simulink model "ex3_3"  (R2021a)
settings: Solver=VariableStepAuto  StartTime=0.0  StopTime=100  RelTol=1e-3
values from neighbouring files (symbols this model uses):
  b = 0.001    [parameters.m]
  D = diag([d,d,d].')    [uas_parameters_mod.m]
  g_acc = 9.81    [parameters.m]    (also in uas_parameters_mod.m)
  I = [Ix 0 0; 0 Iy 0; 0 0 Iz]    [parameters.m]    (also in uas_parameters_mod.m)
  invI = inv(I)    [uas_parameters_mod.m]
  Ix = 3*exp(-3)    [parameters.m]    (also in uas_parameters_mod.m = 3*exp(-6))
  Iy = 3*exp(-3)    [parameters.m]    (also in uas_parameters_mod.m = 3*exp(-6))
  Iz = 5*exp(-6)    [parameters.m]    (also in uas_parameters_mod.m = 1*exp(-5))
  k = 0.01    [parameters.m]
  Kd__y = -0.075*K__y*T__y*45    [uas_parameters_mod.m]
  Kd_p = -0.075*K_p*T_p*17    (= 0.7919025)    [uas_parameters_mod.m]
  Kd_r = -0.075*K_r*T_r*6.2    (= 0.79515)    [uas_parameters_mod.m]
  Kd_x = -0.075*K_x*T_x*45    (= 0.022325972625)    [uas_parameters_mod.m]
  Kd_y = -0.075*K_y*T_y*7    (= 0.937125)    [uas_parameters_mod.m]
  Kd_z = -65    [uas_parameters_mod.m]
  Ki__y = 0    [uas_parameters_mod.m]
  Ki_p = 1.2*K_p/T_p*1.2    (= -0.000231846723555)    [uas_parameters_mod.m]
  Ki_r = 1.2*K_r/T_r*0.3    (= -0.00118421052632)    [uas_parameters_mod.m]
  Ki_y = 1.2*K_y/T_y*0.1    (= -0.000378151260504)    [uas_parameters_mod.m]
  Ki_z = 0.01    [uas_parameters_mod.m]
  Kp__y = 0.6*K__y*15    [uas_parameters_mod.m]
  Kp_p = 0.6*K_p*40    (= -0.24)    [uas_parameters_mod.m]
  Kp_r = 0.6*K_r*6    (= -0.27)    [uas_parameters_mod.m]
  Kp_x = 0.6*K_x*15    (= -0.002097)    [uas_parameters_mod.m]
  Kp_y = 0.6*K_y*10    (= -0.45)    [uas_parameters_mod.m]
  Kp_z = 20    [uas_parameters_mod.m]
  L = 0.225    [parameters.m]    (also in uas_parameters_mod.m)
  m = 0.5    [parameters.m]    (also in uas_parameters_mod.m)
  mg = [0; 0; -m*9.81]    [uas_parameters_mod.m]
libraries: slctrlblks x1, vrlib x1
settings Model: Creator=filippo  LastModifiedBy=filippo

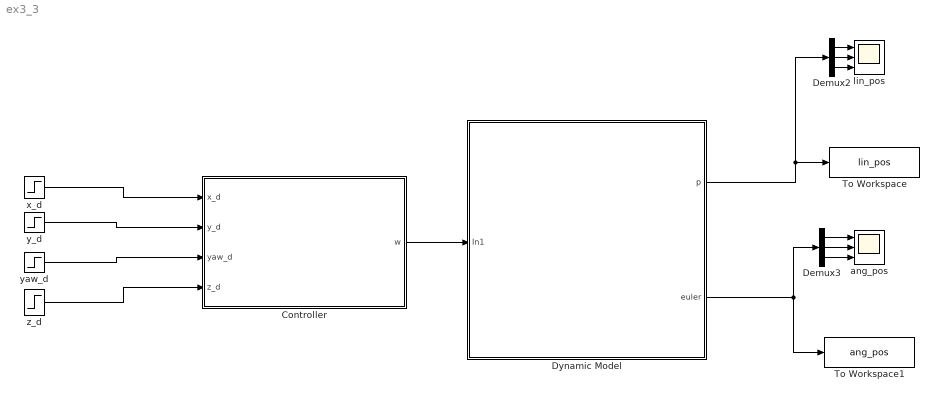
== system ex3_3 ==
  Controller : Subsystem
  Demux2 : Demux  Outputs=3
  Demux3 : Demux  Outputs=3
  Dynamic Model : Subsystem
  To Workspace : ToWorkspace  VariableName=lin_pos  SaveFormat=Timeseries  SampleTime=-1
  To Workspace1 : ToWorkspace  VariableName=ang_pos  SaveFormat=Timeseries  SampleTime=-1
  ang_pos : Scope  NumInputPorts=3
  lin_pos : Scope  NumInputPorts=3
  x_d : Step  SampleTime=0
  y_d : Step  After=0  SampleTime=0
  yaw_d : Step  After=0  SampleTime=0
  z_d : Step  After=0  SampleTime=0
  wires:
  Dynamic Model/2(euler) -> Demux3/1, To Workspace1/1
  Dynamic Model/1(p) -> Demux2/1, To Workspace/1
  Demux2/1 -> lin_pos/1
  Demux3/2 -> ang_pos/2
  Demux2/3 -> lin_pos/3
  Demux2/2 -> lin_pos/2
  Demux3/3 -> ang_pos/3
  Demux3/1 -> ang_pos/1
  Controller/1(w) -> Dynamic Model/1(In1)
  z_d/1 -> Controller/4(z_d)
  x_d/1 -> Controller/1(x_d)
  yaw_d/1 -> Controller/3(yaw_d)
  y_d/1 -> Controller/2(y_d)

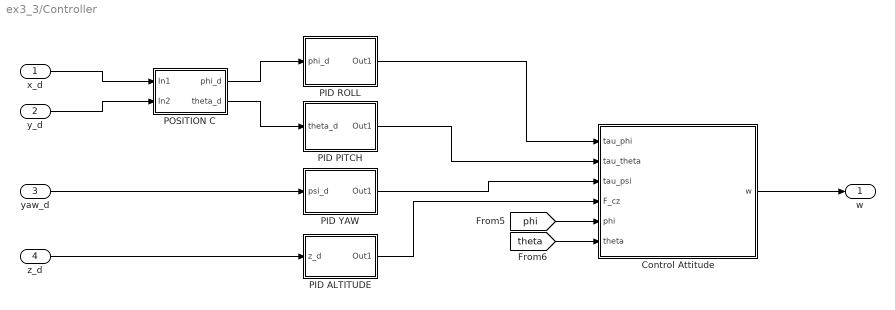
== system ex3_3/Controller ==
  x_d : Inport
  y_d : Inport  Port=2
  yaw_d : Inport  Port=3
  z_d : Inport  Port=4
  Control Attitude : MATLAB Function  TreatAsAtomicUnit=on
  PID ALTITUDE : Subsystem
  PID PITCH : Subsystem
  PID ROLL : Subsystem
  PID YAW : Subsystem
  POSITION C : Subsystem
  w : Outport
  wires:
  PID YAW/1(Out1) -> Control Attitude/3(tau_psi)
  [theta] -> Control Attitude/6(theta)
  PID ROLL/1(Out1) -> Control Attitude/1(tau_phi)
  [phi] -> Control Attitude/5(phi)
  PID ALTITUDE/1(Out1) -> Control Attitude/4(F_cz)
  PID PITCH/1(Out1) -> Control Attitude/2(tau_theta)
  Control Attitude/1(w) -> w/1
  POSITION C/1(phi_d) -> PID ROLL/1(phi_d)
  POSITION C/2(theta_d) -> PID PITCH/1(theta_d)
  x_d/1 -> POSITION C/1(In1)
  y_d/1 -> POSITION C/2(In2)
  z_d/1 -> PID ALTITUDE/1(z_d)
  yaw_d/1 -> PID YAW/1(psi_d)

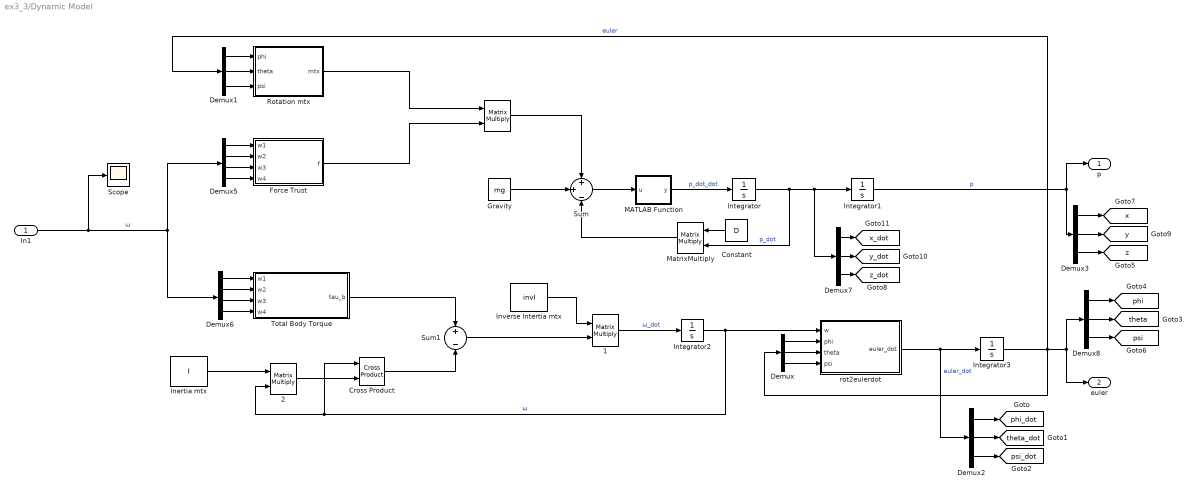
== system ex3_3/Dynamic Model ==
  In1 : Inport
  " " : Product  Multiplication=Matrix(*)
  " 1" : Product  Multiplication=Matrix(*)
  " 2" : Product  Multiplication=Matrix(*)
  Constant : Constant  Value=D
  Cross Product : vrlib/Utilities/Cross Product
  Demux{,1..3,7..8} (6 alike) : Demux  Outputs=3
  Demux5 : Demux
  Demux6 : Demux
  Force Trust : MATLAB Function  TreatAsAtomicUnit=on
  Gravity : Constant  Value=mg  VectorParams1D=off
  Inertia mtx : Constant  Value=I  VectorParams1D=off
  Integrator{,1..3} (4 alike) : Integrator
  Inverse Intertia mtx : Constant  Value=invI
  MATLAB Function : MATLAB Function  TreatAsAtomicUnit=on
  MatrixMultiply : Product  Multiplication=Matrix(*)
  Rotation mtx : MATLAB Function  TreatAsAtomicUnit=on
  Scope : Scope
  Sum : Sum  Inputs=+|+|-
  Sum1 : Sum  Inputs=+|-
  Total Body Torque : MATLAB Function  TreatAsAtomicUnit=on
  rot2eulerdot : MATLAB Function  TreatAsAtomicUnit=on
  p : Outport
  euler : Outport  Port=2
  tag scope: phi=global, phi_dot=global, psi=global, psi_dot=global, theta=global, theta_dot=global, x=global, x_dot=global, y=global, y_dot=global, z=global, z_dot=global
  wires:
  " "/1 -> Sum/1
  Sum/1 -> MATLAB Function/1(u)
  " 2"/1 -> Cross Product/2
  Rotation mtx/1(mtx) -> " "/1
  Demux5/4 -> Force Trust/4(w4)
  Demux1/3 -> Rotation mtx/3(psi)
  Demux5/2 -> Force Trust/2(w2)
  Gravity/1 -> Sum/2
  Demux1/1 -> Rotation mtx/1(phi)
  Demux1/2 -> Rotation mtx/2(theta)
  Demux6/4 -> Total Body Torque/4(w4)
  Demux/2 -> rot2eulerdot/3(theta)
  rot2eulerdot/1(euler_dot) -> Demux2/1, Integrator3/1  "euler_dot"
  Force Trust/1(f) -> " "/2
  Integrator3/1 -> Demux1/1, Demux/1, euler/1, Demux8/1  "euler"
  Demux/1 -> rot2eulerdot/2(phi)
  Demux5/3 -> Force Trust/3(w3)
  Demux6/1 -> Total Body Torque/1(w1)
  In1/1 -> Scope/1, Demux6/1, Demux5/1  "ω"
  Integrator2/1 -> Cross Product/1, " 2"/2, rot2eulerdot/1(w)  "ω"
  Demux6/3 -> Total Body Torque/3(w3)
  Demux/3 -> rot2eulerdot/4(psi)
  Demux5/1 -> Force Trust/1(w1)
  Demux6/2 -> Total Body Torque/2(w2)
  Demux2/1 -> [phi_dot]
  Demux2/3 -> [psi_dot]
  Demux2/2 -> [theta_dot]
  Demux3/3 -> [z]
  Integrator1/1 -> Demux3/1, p/1  "p"
  Integrator/1 -> MatrixMultiply/2, Demux7/1, Integrator1/1  "p_dot"
  Demux7/3 -> [z_dot]
  Demux3/1 -> [x]
  Demux3/2 -> [y]
  Demux7/1 -> [x_dot]
  Demux7/2 -> [y_dot]
  Demux8/1 -> [phi]
  Demux8/2 -> [theta]
  Demux8/3 -> [psi]
  Total Body Torque/1(tau_b) -> Sum1/1
  Cross Product/1 -> Sum1/2
  " 1"/1 -> Integrator2/1  "ω_dot"
  Sum1/1 -> " 1"/2
  Inertia mtx/1 -> " 2"/1
  Inverse Intertia mtx/1 -> " 1"/1
  MATLAB Function/1(y) -> Integrator/1  "p_dot_dot"
  Constant/1 -> MatrixMultiply/1
  MatrixMultiply/1 -> Sum/3

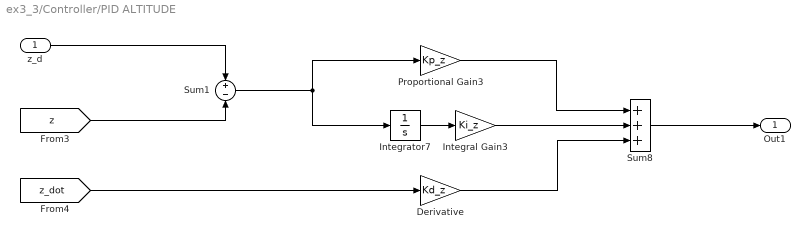
== system ex3_3/Controller/PID ALTITUDE ==
  z_d : Inport
  "Derivative " : Gain  Gain=Kd_z
  Integral Gain3 : Gain  Gain=Ki_z
  Integrator7 : Integrator
  Proportional Gain3 : Gain  Gain=Kp_z
  Sum1 : Sum  Inputs=+|-
  Sum8 : Sum  Inputs=+++
  Out1 : Outport
  wires:
  [z] -> Sum1/2
  "Derivative "/1 -> Sum8/3
  [z_dot] -> "Derivative "/1
  Sum1/1 -> Integrator7/1, Proportional Gain3/1
  Integral Gain3/1 -> Sum8/2
  Integrator7/1 -> Integral Gain3/1
  z_d/1 -> Sum1/1
  Proportional Gain3/1 -> Sum8/1
  Sum8/1 -> Out1/1

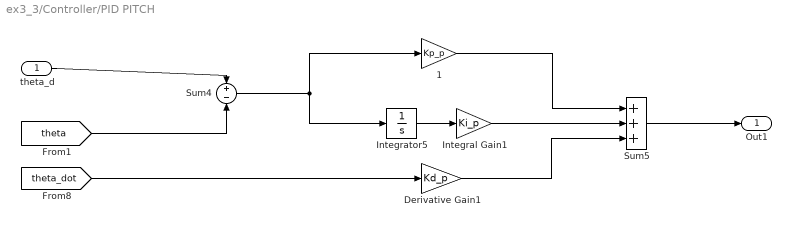
== system ex3_3/Controller/PID PITCH ==
  theta_d : Inport
  " 1" : Gain  Gain=Kp_p
  Derivative Gain1 : Gain  Gain=Kd_p
  Integral Gain1 : Gain  Gain=Ki_p
  Integrator5 : Integrator
  Sum4 : Sum  Inputs=+|-
  Sum5 : Sum  Inputs=+++
  Out1 : Outport
  wires:
  [theta_dot] -> Derivative Gain1/1
  theta_d/1 -> Sum4/1
  Integral Gain1/1 -> Sum5/2
  [theta] -> Sum4/2
  " 1"/1 -> Sum5/1
  Sum4/1 -> " 1"/1, Integrator5/1
  Integrator5/1 -> Integral Gain1/1
  Derivative Gain1/1 -> Sum5/3
  Sum5/1 -> Out1/1

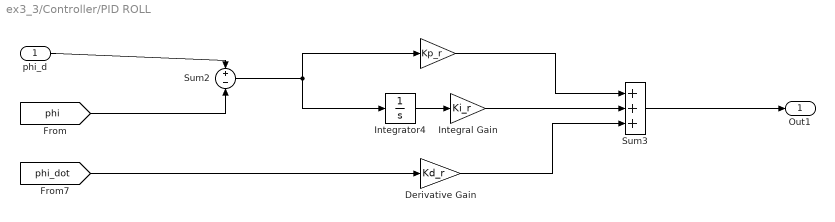
== system ex3_3/Controller/PID ROLL ==
  phi_d : Inport
  " " : Gain  Gain=Kp_r
  Derivative Gain : Gain  Gain=Kd_r
  Integral Gain : Gain  Gain=Ki_r
  Integrator4 : Integrator
  Sum2 : Sum  Inputs=+|-
  Sum3 : Sum  Inputs=+++
  Out1 : Outport
  wires:
  Integrator4/1 -> Integral Gain/1
  phi_d/1 -> Sum2/1
  Sum2/1 -> Integrator4/1, " "/1
  [phi] -> Sum2/2
  [phi_dot] -> Derivative Gain/1
  Derivative Gain/1 -> Sum3/3
  Integral Gain/1 -> Sum3/2
  " "/1 -> Sum3/1
  Sum3/1 -> Out1/1

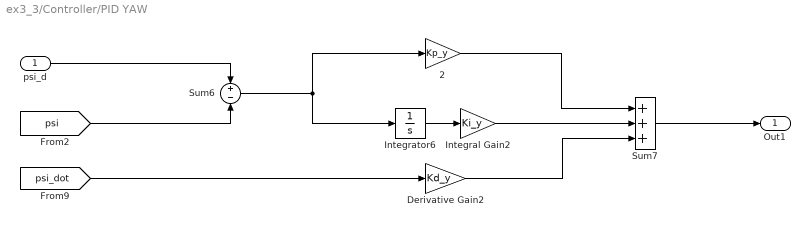
== system ex3_3/Controller/PID YAW ==
  psi_d : Inport
  " 2" : Gain  Gain=Kp_y
  Derivative Gain2 : Gain  Gain=Kd_y
  Integral Gain2 : Gain  Gain=Ki_y
  Integrator6 : Integrator
  Sum6 : Sum  Inputs=+|-
  Sum7 : Sum  Inputs=+++
  Out1 : Outport
  wires:
  [psi_dot] -> Derivative Gain2/1
  Derivative Gain2/1 -> Sum7/3
  psi_d/1 -> Sum6/1
  Integral Gain2/1 -> Sum7/2
  Sum6/1 -> " 2"/1, Integrator6/1
  Sum7/1 -> Out1/1
  [psi] -> Sum6/2
  " 2"/1 -> Sum7/1
  Integrator6/1 -> Integral Gain2/1

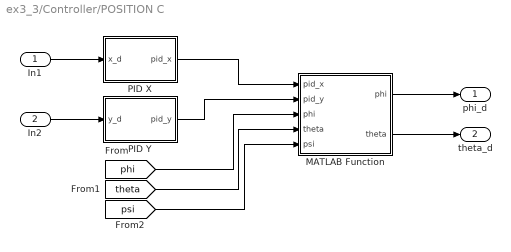
== system ex3_3/Controller/POSITION C ==
  In1 : Inport
  In2 : Inport  Port=2
  MATLAB Function : MATLAB Function  TreatAsAtomicUnit=on
  PID X : Subsystem
  PID Y : Subsystem
  phi_d : Outport
  theta_d : Outport  Port=2
  wires:
  PID X/1(pid_x) -> MATLAB Function/1(pid_x)
  PID Y/1(pid_y) -> MATLAB Function/2(pid_y)
  [phi] -> MATLAB Function/3("phi ")
  [theta] -> MATLAB Function/4("theta ")
  [psi] -> MATLAB Function/5(psi)
  MATLAB Function/1(phi) -> phi_d/1
  MATLAB Function/2(theta) -> theta_d/1
  In1/1 -> PID X/1(x_d)
  In2/1 -> PID Y/1(y_d)

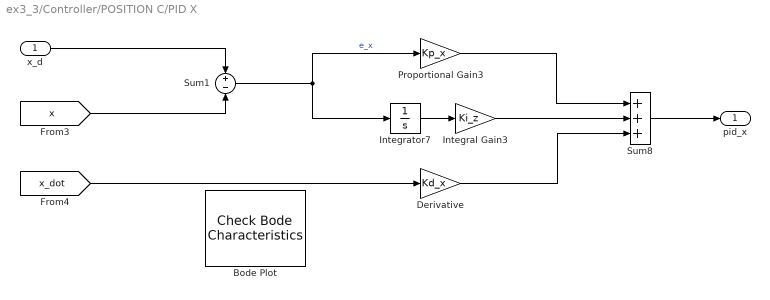
== system ex3_3/Controller/POSITION C/PID X ==
  x_d : Inport
  Bode Plot : slctrlblks/Model Verification/Check Bode  Characteristics  InstantiateOnLoad=on  SaveOperatingPoints=off  LinearizationIOs={'/Controller/POSITION C/PID X/Sum8', 1, 'in', 'off', '';'/Dynamic Model', 1, 'out', 'on', ''}  LinearizeAt=SnapshotTimes  SnapshotTimes=[0]  TriggerType=rising  SampleTime=auto  RateConversionMethod=zoh  PreWarpFreq=10  UseExactDelayModel=off  UseFullBlockNameLabels=off  UseBusSignalLabels=off  enabled=on  stopWhenAssertionFail=off  export=off  ViewDlgPos=[73 1 1848 961]  OpenViewOnLoad=off  LaunchViewOnOpen=off  FrequencyUnits=rad/s  MagnitudeUnits=dB  PhaseUnits=deg  TimeUnits=seconds  EnableUpperBound=off  UpperBoundFrequencies=[]  UpperBoundMagnitudes=[]  EnableLowerBound=off  LowerBoundFrequencies=[]  LowerBoundMagnitudes=[]
      settings: SaveToWorkspace=on
  "Derivative " : Gain  Gain=Kd_x
  Integral Gain3 : Gain  Gain=Ki_z
  Integrator7 : Integrator
  Proportional Gain3 : Gain  Gain=Kp_x
  Sum1 : Sum  Inputs=+|-
  Sum8 : Sum  Inputs=+++
  pid_x : Outport
  wires:
  Sum8/1 -> pid_x/1
  Integral Gain3/1 -> Sum8/2
  [x] -> Sum1/2
  "Derivative "/1 -> Sum8/3
  Sum1/1 -> Integrator7/1, Proportional Gain3/1  "e_x"
  [x_dot] -> "Derivative "/1
  Integrator7/1 -> Integral Gain3/1
  Proportional Gain3/1 -> Sum8/1
  x_d/1 -> Sum1/1

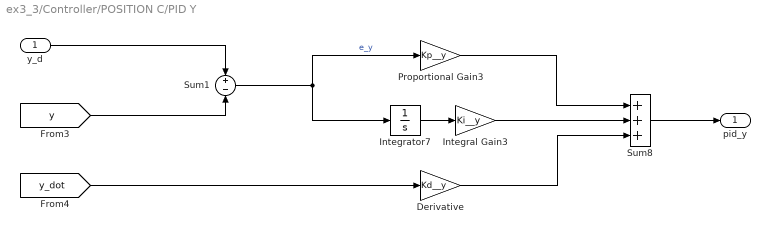
== system ex3_3/Controller/POSITION C/PID Y ==
  y_d : Inport
  "Derivative " : Gain  Gain=Kd__y
  Integral Gain3 : Gain  Gain=Ki__y
  Integrator7 : Integrator
  Proportional Gain3 : Gain  Gain=Kp__y
  Sum1 : Sum  Inputs=+|-
  Sum8 : Sum  Inputs=+++
  pid_y : Outport
  wires:
  Sum8/1 -> pid_y/1
  Integral Gain3/1 -> Sum8/2
  [y] -> Sum1/2
  "Derivative "/1 -> Sum8/3
  Sum1/1 -> Integrator7/1, Proportional Gain3/1  "e_y"
  [y_dot] -> "Derivative "/1
  Integrator7/1 -> Integral Gain3/1
  Proportional Gain3/1 -> Sum8/1
  y_d/1 -> Sum1/1

== matlab function ex3_3/Dynamic Model/Force Trust ==
  data: w1 input; f output [..2]; w2 input; w3 input; w4 input; k parameter
function f = F_b(w1,w2,w3,w4,k)
mtx = k*[0; 0; w1+w2+w3+w4];
f = mtx;
end

== matlab function ex3_3/Dynamic Model/Rotation mtx ==
  data: phi input; mtx output; theta input; psi input
function mtx = ROTATION(phi, theta, psi)
Rx = [1 0 0; 
      0 cos(phi) -sin(phi); 
      0 sin(phi) cos(phi)];
Ry = [cos(theta) 0 sin(theta); 
      0 1 0; 
      -sin(theta) 0 cos(theta)];
Rz = [cos(psi) -sin(psi) 0; 
      sin(psi) cos(psi) 0; 
      0 0 1];

% Rot matrix Body-fixed frame wrt Inertial frame
R = Rz * Ry * Rx;
mtx = R;
end

== matlab function ex3_3/Dynamic Model/Total Body Torque ==
  data: w1 input; tau_b output; w2 input; w3 input; w4 input; L parameter; k parameter; b parameter
function tau_b= TotalBodyTorque(w1, w2, w3, w4, L, k, b)
tau_b = [L*k*(w1-w3);
         L*k*(w2-w4); 
         b*(w1-w2+w3-w4)];
end

== matlab function ex3_3/Dynamic Model/MATLAB Function ==
  data: u input; y output; M parameter
function y = fcn(u, M)
invM = inv(M);
y = invM*u;
end

== matlab function ex3_3/Dynamic Model/rot2eulerdot ==
  data: w input; phi input; euler_dot output; theta input; psi input
function euler_dot = rot2euler(w, phi, theta, psi)
R = [1 0 -sin(theta); 
     0 cos(phi) cos(theta)*sin(phi);
     0 -sin(phi) cos(theta)*cos(phi)];
invR = inv(R);
euler_dot = invR*w;
end

== matlab function ex3_3/Controller/Control Attitude ==
  data: tau_phi input; w output; tau_theta input; tau_psi input; F_cz input; phi input; theta input; Ix parameter; Iy parameter; Iz parameter; L parameter; k parameter; b parameter; m parameter; g_acc parameter
function w = AttitudeControl(tau_phi, tau_theta, tau_psi,F_cz, phi, theta, Ix, Iy, Iz, L, k, b, m, g_acc)
A = [L*k 0 -L*k 0;
     0 L*k 0 -L*k;
     b -b b -b;
     1 1 1 1];
inv_A = inv(A);
U = [-Ix*tau_phi;
     -Iy*tau_theta;
     -Iz*tau_psi;
     m*g_acc/(k*cos(theta)*cos(phi)) + F_cz];
w = inv_A*U;
end

== matlab function ex3_3/Controller/POSITION C/MATLAB Function ==
  data: pid_x input; phi output; pid_y input; phi input; theta input; psi input; theta output
function [phi, theta] = fcn(pid_x, pid_y, phi, theta, psi)
Rx = [1 0 0; 
      0 cos(phi) -sin(phi); 
      0 sin(phi) cos(phi)];
Ry = [cos(theta) 0 sin(theta); 
      0 1 0; 
      -sin(theta) 0 cos(theta)];
Rz = [cos(psi) -sin(psi) 0; 
      sin(psi) cos(psi) 0; 
      0 0 1];
% Rot matrix Body-fixed frame wrt Inertial frame
R = Rz * Ry * Rx;

mtx = [0 1 0; -1 0 0];

PID = [pid_x; pid_y; 0];

A = mtx*R*PID;
phi = A(1,1);
theta = A(2,1);
end
